simulink model "javi_FULL_model"  (R2023a)
settings: Solver=VariableStepAuto  StartTime=0.0  StopTime=0.5  RelTol=1e-3
undefined symbols (not defined in the file or in its folder): f_grid, L, R, tau, Vpeak_d1
libraries: spsControlledVoltageSourceLib x6, slpidlib x4, spsCurrentMeasurementLib x3, spsSeriesRLCBranchLib x3, powerlib_extras x1, spspowerguiLib x1
settings Model: Creator=citcea  LastModifiedBy=citcea

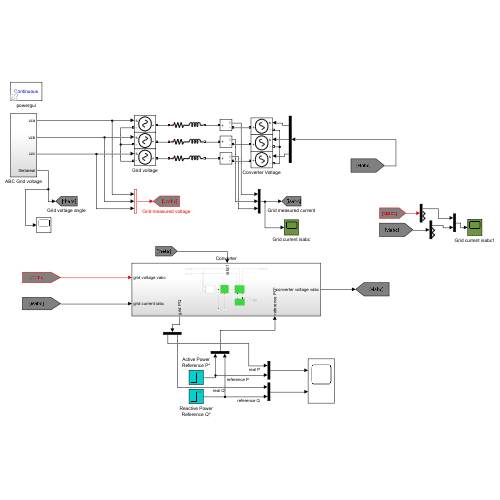
[thumbnail: Simulink's stored preview of the top-level diagram]
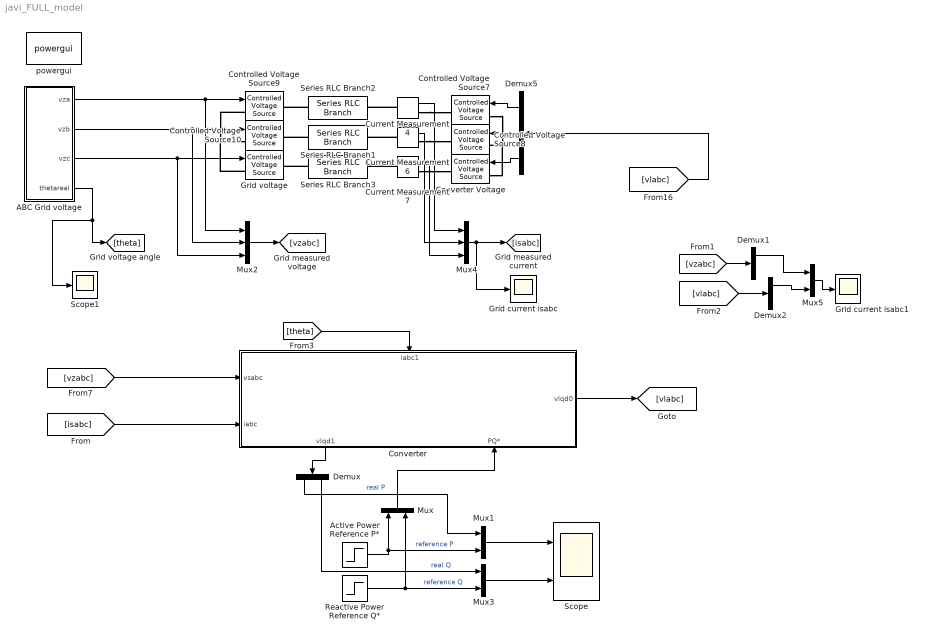
== system javi_FULL_model ==
  ABC Grid voltage : Subsystem
  Active Power Reference P* : Step  Time=0.1  After=100e6  SampleTime=0
  Controlled Voltage Source{7..10} (4 alike) : spsControlledVoltageSourceLib/Controlled Voltage Source  Initialize=off  Source_Type=AC  Amplitude=0  Phase=0  Frequency=0  Measurements=None
  Converter : Subsystem
      settings: PortSchema="{\"entries\":[{\"content\":{\"sides\":[{\"content\":{\"connectorIds\":[\"In1\",\"In2\"]},\"type\":\"ConnectorPlacement.EquallySpacedRectSide\",\"uuid\":\"584062e5-d349-4a6c-b774-2e2a2bb48d68\"},{\"content\":{\"connectorIds\":[\"Out1\"],\"side\":\"RIGHT\"},\"type\":\"ConnectorPlacement.EquallySpacedRectSide\",\"uuid\":\"a9b3d7e8-76a4-441e-96b8-94fa9e4298b7\"},{\"content\":{\"connectorIds\":[\"In3\"],\"side\":\"TOP\"},\"type\":\"ConnectorPlacement.EquallySpacedRectSide\",\"uuid\":\"fa132551-d5a3-4871-9f18-bb1732292fbb\"},{\"content\":{\"connectorIds\":[\"Out2\",\"In4\"],\"side\":\"BOTTOM\"},\"type\":\"ConnectorPlacement.EquallySpacedRectSide\",\"uuid\":\"9abb25d7-96ea-4765-9339-f819af1c9234\"}]},\"type\":\"ConnectorPlacement.EquallySpacedConnector\",\"uuid\":\"67c0bfb2-b216-417e-864f-4c59b5de7996\"}],\"packageUris\":[\"http://schema.mathworks.com/mf0/Connector/R2020b\"],\"version\":\"1.0\"}"
  Converter Voltage : spsControlledVoltageSourceLib/Controlled Voltage Source  Initialize=off  Source_Type=AC  Amplitude=0  Phase=0  Frequency=0  Measurements=None
  Current Measurement4 : spsCurrentMeasurementLib/Current Measurement  PhasorSimulation=off  OutputType=Complex  PSBequivalent=0
  Current Measurement6 : spsCurrentMeasurementLib/Current Measurement  PhasorSimulation=off  OutputType=Complex  PSBequivalent=0
  Current Measurement7 : spsCurrentMeasurementLib/Current Measurement  PhasorSimulation=off  OutputType=Complex  PSBequivalent=0
  Demux : Demux  Outputs=2
  Demux1 : Demux  Outputs=3
  Demux2 : Demux  Outputs=3
  Demux5 : Demux  Outputs=3
  Grid current isabc : Scope
  Grid current isabc1 : Scope
  Grid voltage : spsControlledVoltageSourceLib/Controlled Voltage Source  Initialize=off  Source_Type=AC  Amplitude=0  Phase=0  Frequency=0  Measurements=None
  Mux{,1,3,5} (4 alike) : Mux  Inputs=2
  Mux2 : Mux  Inputs=3
  Mux4 : Mux  Inputs=3
  Reactive Power Reference Q* : Step  Time=0.3  After=10e6  SampleTime=0
  Scope : Scope  NumInputPorts=2
  Scope1 : Scope
  Series RLC Branch1 : spsSeriesRLCBranchLib/Series RLC Branch  LConnTagsString=__new0  RConnTagsString=__new0  BranchType=RL  Resistance=R  Inductance=L  SetiL0=off  InitialCurrent=0  Capacitance=0  Setx0=off  InitialVoltage=0  Measurements=None
  Series RLC Branch2 : spsSeriesRLCBranchLib/Series RLC Branch  LConnTagsString=__new0  RConnTagsString=__new0  BranchType=RL  Resistance=R  Inductance=L  SetiL0=off  InitialCurrent=0  Capacitance=0  Setx0=off  InitialVoltage=0  Measurements=None
  Series RLC Branch3 : spsSeriesRLCBranchLib/Series RLC Branch  LConnTagsString=__new0  RConnTagsString=__new0  BranchType=RL  Resistance=R  Inductance=L  SetiL0=off  InitialCurrent=0  Capacitance=0  Setx0=off  InitialVoltage=0  Measurements=None
  powergui : spspowerguiLib/powergui  Priority=1  SimulationMode=Continuous  SampleTime=50e-6  frequency=60  Iterations=50  frequencyindice=0  Pbase=100e6  ErrMax=1e-4  UnitsV=kV  UnitsW=MW  buscounter=0  FunctionMessages=off  echomessages=off  EnableUseOfTLC=off  CurrentSourceSwitches=on  DisableSnubberDevices=off  DisableRonSwitches=off  DisableVfSwitches=off  DisplayEquations=off  AutomaticDiscreteSolvers=off  SolverType=Tustin  Interpol=off  ExternalGateDelay=off  methode=off  Ts=0  x0status=blocks  SPID=off  SwTol=0  HookPort=off  NonlinearTolerance=1e-4  nMaxIteration=100  ContinueOnMaxIteration=off  RestoreLinks=warning  ResistiveCurrentMeasurement=off  Frange=[0:2:500]  Ylog=off  Xlog=on  ShowGrid=off  save=off  variable=ZData  structure=0  ZoomFFT=off  StartTime=0.0  cycles=1  DisplayStyle=1  fundamental=60  FreqAxis=off  MaxFrequency=1000  frequencyindicesteady=1  RmsSteady=1  display=off
  wires:
  Mux2/1 -> [vzabc]
  Current Measurement4/1 -> Mux4/1
  Current Measurement6/1 -> Mux4/2
  Mux4/1 -> [isabc], Grid current isabc/1
  Current Measurement7/1 -> Mux4/3
  Demux5/3 -> Converter Voltage/1
  Demux5/1 -> Controlled Voltage Source7/1
  ABC Grid voltage/1(vza) -> Controlled Voltage Source9/1, Mux2/1
  ABC Grid voltage/2(vzb) -> Controlled Voltage Source10/1, Mux2/2
  ABC Grid voltage/3(vzc) -> Grid voltage/1, Mux2/3
  [vlabc] -> Demux5/1
  Demux5/2 -> Controlled Voltage Source8/1
  ABC Grid voltage/4(thetareal) -> Scope1/1, [theta]
  Converter/1(vlqd0) -> [vlabc]
  [isabc] -> Converter/2(iabc)
  [vzabc] -> Converter/1(vsabc)
  Mux/1 -> Converter/4(PQ*)
  Active Power Reference P*/1 -> Mux1/2, Mux/1  "reference P"
  Reactive Power Reference Q*/1 -> Mux3/2, Mux/2  "reference Q"
  Converter/2(vlqd1) -> Demux/1
  Demux/1 -> Mux1/1  "real P"
  Mux1/1 -> Scope/1
  Mux3/1 -> Scope/2
  Demux/2 -> Mux3/1  "real Q"
  [vzabc] -> Demux1/1
  [vlabc] -> Demux2/1
  Demux1/1 -> Mux5/1
  Mux5/1 -> Grid current isabc1/1
  Demux2/1 -> Mux5/2
  [theta] -> Converter/3(iabc1)
  connections:
  Grid voltage/LConn1 -- Controlled Voltage Source9/LConn1 -- Controlled Voltage Source10/LConn1
  Converter Voltage/LConn1 -- Controlled Voltage Source7/LConn1 -- Controlled Voltage Source8/LConn1
  Current Measurement4/LConn1 -- Series RLC Branch2/RConn1
  Series RLC Branch1/LConn1 -- Controlled Voltage Source10/RConn1
  Current Measurement6/RConn1 -- Controlled Voltage Source8/RConn1
  Current Measurement7/LConn1 -- Series RLC Branch3/RConn1
  Series RLC Branch2/LConn1 -- Controlled Voltage Source9/RConn1
  Current Measurement4/RConn1 -- Controlled Voltage Source7/RConn1
  Current Measurement6/LConn1 -- Series RLC Branch1/RConn1
  Current Measurement7/RConn1 -- Converter Voltage/RConn1
  Series RLC Branch3/LConn1 -- Grid voltage/RConn1

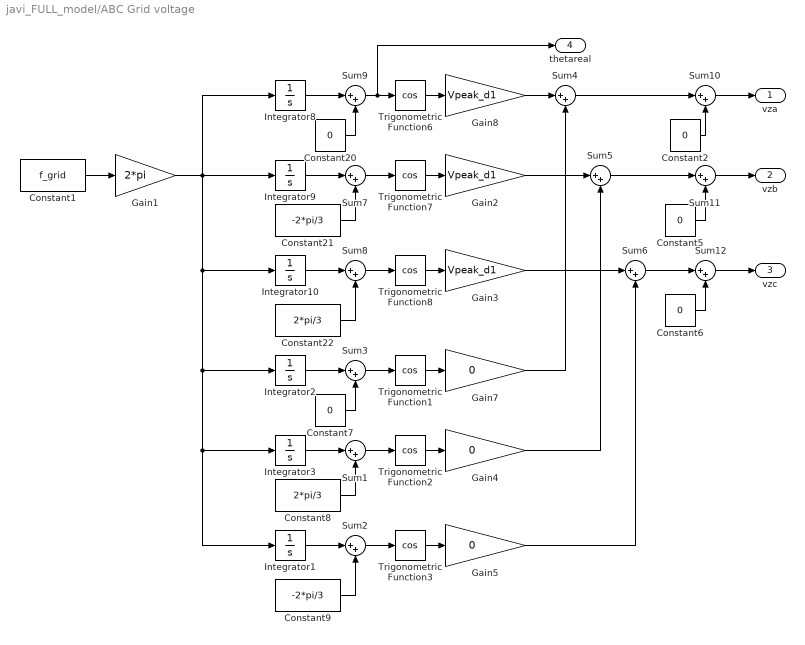
== system javi_FULL_model/ABC Grid voltage ==
  Constant1 : Constant  Value=f_grid
  Constant{2,5..7,20} (5 alike) : Constant  Value=0
  Constant21 : Constant  Value=-2*pi/3
  Constant22 : Constant  Value=2*pi/3
  Constant8 : Constant  Value=2*pi/3
  Constant9 : Constant  Value=-2*pi/3
  Gain1 : Gain  Gain=2*pi
  Gain2 : Gain  Gain=Vpeak_d1
  Gain3 : Gain  Gain=Vpeak_d1
  Gain4 : Gain  Gain=0
  Gain5 : Gain  Gain=0
  Gain7 : Gain  Gain=0
  Gain8 : Gain  Gain=Vpeak_d1
  Integrator{1..3,8..10} (6 alike) : Integrator
  Sum{1..12} (12 alike) : Sum  Inputs=|++
  Trigonometric Function{1..3,6..8} (6 alike) : Trigonometry  Operator=cos
  vza : Outport
  vzb : Outport  Port=2
  vzc : Outport  Port=3
  thetareal : Outport  Port=4
  wires:
  Sum12/1 -> vzc/1
  Sum11/1 -> vzb/1
  Sum10/1 -> vza/1
  Constant6/1 -> Sum12/2
  Constant5/1 -> Sum11/2
  Constant2/1 -> Sum10/2
  Sum6/1 -> Sum12/1
  Sum5/1 -> Sum11/1
  Sum4/1 -> Sum10/1
  Gain5/1 -> Sum6/2
  Gain4/1 -> Sum5/2
  Gain7/1 -> Sum4/2
  Trigonometric Function2/1 -> Gain4/1
  Trigonometric Function3/1 -> Gain5/1
  Sum3/1 -> Trigonometric Function1/1
  Constant9/1 -> Sum2/2
  Integrator1/1 -> Sum2/1
  Constant8/1 -> Sum1/2
  Integrator2/1 -> Sum3/1
  Gain1/1 -> Integrator9/1, Integrator8/1, Integrator10/1, Integrator2/1, Integrator1/1, Integrator3/1
  Sum1/1 -> Trigonometric Function2/1
  Constant7/1 -> Sum3/2
  Trigonometric Function1/1 -> Gain7/1
  Integrator3/1 -> Sum1/1
  Sum2/1 -> Trigonometric Function3/1
  Gain3/1 -> Sum6/1
  Gain2/1 -> Sum5/1
  Gain8/1 -> Sum4/1
  Trigonometric Function7/1 -> Gain2/1
  Trigonometric Function8/1 -> Gain3/1
  Constant1/1 -> Gain1/1
  Sum9/1 -> thetareal/1, Trigonometric Function6/1
  Constant22/1 -> Sum8/2
  Integrator10/1 -> Sum8/1
  Constant21/1 -> Sum7/2
  Integrator8/1 -> Sum9/1
  Sum7/1 -> Trigonometric Function7/1
  Constant20/1 -> Sum9/2
  Trigonometric Function6/1 -> Gain8/1
  Integrator9/1 -> Sum7/1
  Sum8/1 -> Trigonometric Function8/1

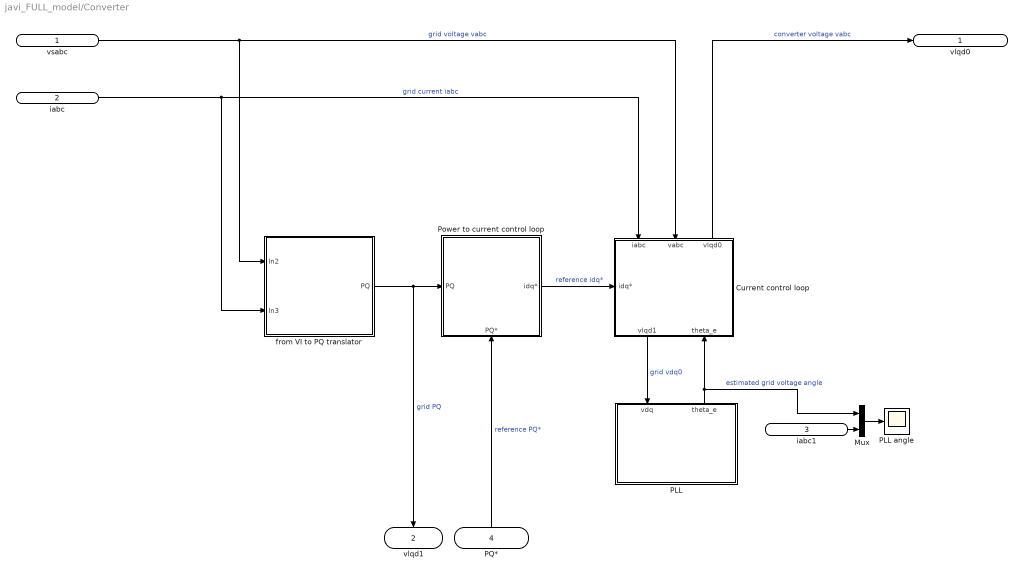
== system javi_FULL_model/Converter ==
  vsabc : Inport
  iabc : Inport  Port=2
  iabc1 : Inport  Port=3
  PQ* : Inport  Port=4
  Current control loop : Subsystem
      settings: PortSchema="{\"entries\":[{\"content\":{\"sides\":[{\"content\":{\"connectorIds\":[\"Out2\",\"In1\",\"In2\"]},\"type\":\"ConnectorPlacement.EquallySpacedRectSide\",\"uuid\":\"c04b464b-16ba-43bf-8c89-b835a7ede4b9\"},{\"content\":{\"connectorIds\":[\"In4\",\"Out1\"],\"side\":\"RIGHT\"},\"type\":\"ConnectorPlacement.EquallySpacedRectSide\",\"uuid\":\"740409c7-44aa-4313-af5e-f03563efb312\"},{\"content\":{\"side\":\"TOP\"},\"type\":\"ConnectorPlacement.EquallySpacedRectSide\",\"uuid\":\"d5fc34f0-88c0-4064-a212-e2f3525e0a41\"},{\"content\":{\"connectorIds\":[\"In3\"],\"side\":\"BOTTOM\"},\"type\":\"ConnectorPlacement.EquallySpacedRectSide\",\"uuid\":\"00c4ea66-ebf3-4884-86d2-74a5a00dfdcd\"}]},\"type\":\"ConnectorPlacement.EquallySpacedConnector\",\"uuid\":\"5b1879ce-fc34-4228-81c6-be4d14a0039a\"}],\"packageUris\":[\"http://schema.mathworks.com/mf0/Connector/R2020b\"],\"version\":\"1.0\"}"
  Mux : Mux  Inputs=2
  PLL : Subsystem
      settings: PortSchema="{\"entries\":[{\"content\":{\"sides\":[{\"content\":{\"connectorIds\":[\"Out1\",\"In1\"]},\"type\":\"ConnectorPlacement.EquallySpacedRectSide\",\"uuid\":\"1b368b75-2a8e-4f20-b703-977c9b032793\"},{\"content\":{\"side\":\"RIGHT\"},\"type\":\"ConnectorPlacement.EquallySpacedRectSide\",\"uuid\":\"82ee01ed-1d9e-40c1-8ec1-273e9e3bb456\"},{\"content\":{\"side\":\"TOP\"},\"type\":\"ConnectorPlacement.EquallySpacedRectSide\",\"uuid\":\"dfdc63e3-35c4-4b8d-aa5d-f501c13e42c1\"}]},\"type\":\"ConnectorPlacement.EquallySpacedConnector\",\"uuid\":\"13f018e6-0609-4dc5-a634-49aff68fea1b\"}],\"packageUris\":[\"http://schema.mathworks.com/mf0/Connector/R2020b\"],\"version\":\"1.0\"}"
  PLL angle : Scope
  Power to current control loop : Subsystem
      settings: PortSchema="{\"entries\":[{\"content\":{\"sides\":[{\"content\":{},\"type\":\"ConnectorPlacement.EquallySpacedRectSide\",\"uuid\":\"ef825e86-9abb-4c1d-b219-2a192ab282df\"},{\"content\":{\"connectorIds\":[\"In2\"],\"side\":\"RIGHT\"},\"type\":\"ConnectorPlacement.EquallySpacedRectSide\",\"uuid\":\"034459b8-9f08-4096-b542-16491f7ea4b2\"},{\"content\":{\"connectorIds\":[\"Out1\"],\"side\":\"TOP\"},\"type\":\"ConnectorPlacement.EquallySpacedRectSide\",\"uuid\":\"d0060c23-b394-4ccb-8e17-1dfe8e516f04\"},{\"content\":{\"connectorIds\":[\"In1\"],\"side\":\"BOTTOM\"},\"type\":\"ConnectorPlacement.EquallySpacedRectSide\",\"uuid\":\"50af44c6-d361-47aa-a23f-971b5daa1a8c\"}]},\"type\":\"ConnectorPlacement.EquallySpacedConnector\",\"uuid\":\"aefb8199-1196-4dbb-bffd-0cb2c3c781ab\"}],\"packageUris\":[\"http://schema.mathworks.com/mf0/Connector/R2020b\"],\"version\":\"1.0\"}"
  from VI to PQ translator : Subsystem
  vlqd0 : Outport
  vlqd1 : Outport  Port=2
  wires:
  vsabc/1 -> Current control loop/1(vabc), from VI to PQ translator/1(In2)  "grid voltage vabc"
  iabc/1 -> Current control loop/2(iabc), from VI to PQ translator/2(In3)  "grid current iabc"
  Current control loop/2(vlqd0) -> vlqd0/1  "converter voltage vabc"
  PLL/1(theta_e) -> Mux/1, Current control loop/4(theta_e)  "estimated grid voltage angle"
  Power to current control loop/1(idq*) -> Current control loop/3(idq*)  "reference idq*"
  PQ*/1 -> Power to current control loop/2(PQ*)  "reference PQ*"
  from VI to PQ translator/1(PQ) -> Power to current control loop/1(PQ), vlqd1/1  "grid PQ"
  Current control loop/1(vlqd1) -> PLL/1(vdq)  "grid vdq0"
  iabc1/1 -> Mux/2
  Mux/1 -> PLL angle/1

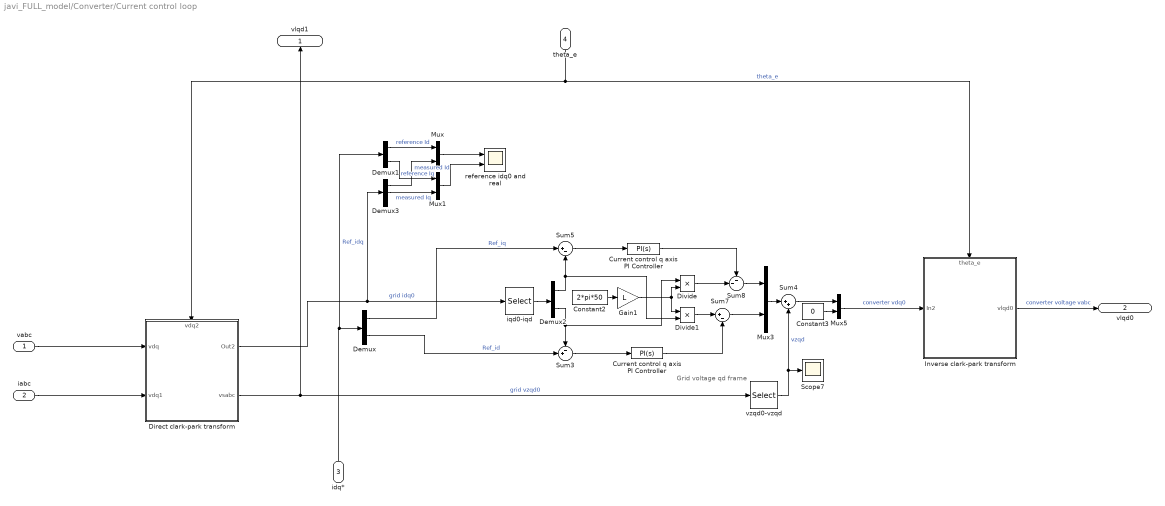
== system javi_FULL_model/Converter/Current control loop ==
  note: Grid voltage qd frame
  vabc : Inport
  iabc : Inport  Port=2
  idq* : Inport  Port=3
  theta_e : Inport  Port=4
  Constant2 : Constant  Value=2*pi*50  SampleTime=-1
  Constant3 : Constant  Value=0
  Current control q axis PI Controller : slpidlib/PID Controller  Controller=PI  Form=Parallel  TimeDomain=Continuous-time  UseExternalTs=off  SampleTime=1  IntegratorMethod=Forward Euler  FilterMethod=Forward Euler  ControllerParametersSource=internal  P=L/tau  I=R/tau  UseKiTs=off  D=0  N=100  UseFilter=on  TunerSelectOption=Transfer Function Based (PID Tuner App)  InitialConditionSource=internal  InitialConditionForIntegrator=0  InitialConditionForFilter=0  DifferentiatorICPrevScaledInput=0  ExternalReset=none  TrackingMode=off  Kt=1  LimitOutput=off  SatLimitsSource=internal  UpperSaturationLimit=inf  LowerSaturationLimit=-inf  LinearizeAsGain=on  AntiWindupMode=none  Kb=1  LimitIntegrator=off  UpperIntegratorSaturationLimit=inf  LowerIntegratorSaturationLimit=-inf  POutMin=[]  POutMax=[]  IOutMin=[]  IOutMax=[]  DOutMin=[]  DOutMax=[]  NOutMin=[]  NOutMax=[]  SumOutMin=[]  SumOutMax=[]  SaturationOutMin=[]  SaturationOutMax=[]  PParamMin=[]  PParamMax=[]  IParamMin=[]  IParamMax=[]  DParamMin=[]  DParamMax=[]  NParamMin=[]  NParamMax=[]  KbParamMin=[]  KbParamMax=[]  KtParamMin=[]  KtParamMax=[]  KbOutMin=[]  KbOutMax=[]  KtOutMin=[]  KtOutMax=[]  IntegratorOutMin=[]  IntegratorOutMax=[]  FilterOutMin=[]  FilterOutMax=[]  SumI1OutMin=[]  SumI1OutMax=[]  SumI2OutMin=[]  SumI2OutMax=[]  SumI3OutMin=[]  SumI3OutMax=[]  SumI4OutMin=[]  SumI4OutMax=[]  SumDOutMin=[]  SumDOutMax=[]  DifferentiatorOutMin=[]  DifferentiatorOutMax=[]  FilterDiffOutCoefMin=[]  FilterDiffOutCoefMax=[]  ReciprocalOutMin=[]  ReciprocalOutMax=[]  SumDenOutMin=[]  SumDenOutMax=[]  SumNumOutMin=[]  SumNumOutMax=[]  DivideOutMin=[]  DivideOutMax=[]  UdiffTsProdOutMin=[]  UdiffTsProdOutMax=[]  NTsProdOutMin=[]  NTsProdOutMax=[]  UintegralTsProdOutMin=[]  UintegralTsProdOutMax=[]  UngainTsProdOutMin=[]  UngainTsProdOutMax=[]  ClampingZeroOutDataTypeStr=Inherit: Inherit via back propagation  ClampingZeroOutMin=[]  ClampingZeroOutMax=[]  FilterDenConstantOutDataTypeStr=Inherit: Inherit via back propagation  FilterDenConstantOutMin=[]  FilterDenConstantOutMax=[]  PCopyOutDataTypeStr=Inherit: Inherit via back propagation  PCopyOutMin=[]  PCopyOutMax=[]  NCopyOutDataTypeStr=Inherit: Inherit via back propagation  NCopyOutMin=[]  NCopyOutMax=[]  IntegratorContinuousStateAttributes=''  IntegratorStateMustResolveToSignalObject=off  IntegratorRTWStateStorageClass=Auto  FilterContinuousStateAttributes=''  FilterStateMustResolveToSignalObject=off  FilterRTWStateStorageClass=Auto  ParallelPVariant=InternalParameters  IdealPVariant=Disabled  IVariant=InternalParameters  DVariant=Disabled  IntegratorVariant=Continuous  SatVariant=Disabled  AWVariant=Passthrough  PCopyVariant=Disabled  TRVariant=Disabled  FdbkBlocksVariant=Forward  IdealPFdbkVariant=Disabled  SatFdbkVariant=Disabled  DerivativeFilterVariant=Disabled  NVariant=Disabled  NCopyVariant=Disabled_SignalSpec  FilterICVariant=Disabled  IntegratorICVariant=InternalICs  ExternalResetVariant=Disabled  TRSumVariant=Passthrough  SumFdbkVariant=Disabled  SumVariant=Sum_PI  TsampFilterVariant=InternalTs  TsampNgainVariant=Passthrough  TsampIntegralVariant=Disabled_SignalSpec  ExternalSaturationOutDataTypeStr=Inherit: Same as second input
  "Current control q axis PI Controller " : slpidlib/PID Controller  Controller=PI  Form=Parallel  TimeDomain=Continuous-time  UseExternalTs=off  SampleTime=1  IntegratorMethod=Forward Euler  FilterMethod=Forward Euler  ControllerParametersSource=internal  P=L/tau  I=R/tau  UseKiTs=off  D=0  N=100  UseFilter=on  TunerSelectOption=Transfer Function Based (PID Tuner App)  InitialConditionSource=internal  InitialConditionForIntegrator=0  InitialConditionForFilter=0  DifferentiatorICPrevScaledInput=0  ExternalReset=none  TrackingMode=off  Kt=1  LimitOutput=off  SatLimitsSource=internal  UpperSaturationLimit=inf  LowerSaturationLimit=-inf  LinearizeAsGain=on  AntiWindupMode=none  Kb=1  LimitIntegrator=off  UpperIntegratorSaturationLimit=inf  LowerIntegratorSaturationLimit=-inf  POutMin=[]  POutMax=[]  IOutMin=[]  IOutMax=[]  DOutMin=[]  DOutMax=[]  NOutMin=[]  NOutMax=[]  SumOutMin=[]  SumOutMax=[]  SaturationOutMin=[]  SaturationOutMax=[]  PParamMin=[]  PParamMax=[]  IParamMin=[]  IParamMax=[]  DParamMin=[]  DParamMax=[]  NParamMin=[]  NParamMax=[]  KbParamMin=[]  KbParamMax=[]  KtParamMin=[]  KtParamMax=[]  KbOutMin=[]  KbOutMax=[]  KtOutMin=[]  KtOutMax=[]  IntegratorOutMin=[]  IntegratorOutMax=[]  FilterOutMin=[]  FilterOutMax=[]  SumI1OutMin=[]  SumI1OutMax=[]  SumI2OutMin=[]  SumI2OutMax=[]  SumI3OutMin=[]  SumI3OutMax=[]  SumI4OutMin=[]  SumI4OutMax=[]  SumDOutMin=[]  SumDOutMax=[]  DifferentiatorOutMin=[]  DifferentiatorOutMax=[]  FilterDiffOutCoefMin=[]  FilterDiffOutCoefMax=[]  ReciprocalOutMin=[]  ReciprocalOutMax=[]  SumDenOutMin=[]  SumDenOutMax=[]  SumNumOutMin=[]  SumNumOutMax=[]  DivideOutMin=[]  DivideOutMax=[]  UdiffTsProdOutMin=[]  UdiffTsProdOutMax=[]  NTsProdOutMin=[]  NTsProdOutMax=[]  UintegralTsProdOutMin=[]  UintegralTsProdOutMax=[]  UngainTsProdOutMin=[]  UngainTsProdOutMax=[]  ClampingZeroOutDataTypeStr=Inherit: Inherit via back propagation  ClampingZeroOutMin=[]  ClampingZeroOutMax=[]  FilterDenConstantOutDataTypeStr=Inherit: Inherit via back propagation  FilterDenConstantOutMin=[]  FilterDenConstantOutMax=[]  PCopyOutDataTypeStr=Inherit: Inherit via back propagation  PCopyOutMin=[]  PCopyOutMax=[]  NCopyOutDataTypeStr=Inherit: Inherit via back propagation  NCopyOutMin=[]  NCopyOutMax=[]  IntegratorContinuousStateAttributes=''  IntegratorStateMustResolveToSignalObject=off  IntegratorRTWStateStorageClass=Auto  FilterContinuousStateAttributes=''  FilterStateMustResolveToSignalObject=off  FilterRTWStateStorageClass=Auto  ParallelPVariant=InternalParameters  IdealPVariant=Disabled  IVariant=InternalParameters  DVariant=Disabled  IntegratorVariant=Continuous  SatVariant=Disabled  AWVariant=Passthrough  PCopyVariant=Disabled  TRVariant=Disabled  FdbkBlocksVariant=Forward  IdealPFdbkVariant=Disabled  SatFdbkVariant=Disabled  DerivativeFilterVariant=Disabled  NVariant=Disabled  NCopyVariant=Disabled_SignalSpec  FilterICVariant=Disabled  IntegratorICVariant=InternalICs  ExternalResetVariant=Disabled  TRSumVariant=Passthrough  SumFdbkVariant=Disabled  SumVariant=Sum_PI  TsampFilterVariant=InternalTs  TsampNgainVariant=Passthrough  TsampIntegralVariant=Disabled_SignalSpec  ExternalSaturationOutDataTypeStr=Inherit: Same as second input
  Demux : Demux  Outputs=2
  Demux1 : Demux  Outputs=2
  Demux2 : Demux  Outputs=2
  Demux3 : Demux  Outputs=3
  Direct clark-park transform : Subsystem
      settings: PortSchema="{\"entries\":[{\"content\":{\"sides\":[{\"content\":{\"connectorIds\":[\"In1\",\"In2\"]},\"type\":\"ConnectorPlacement.EquallySpacedRectSide\",\"uuid\":\"fbcb26c8-642f-4dfe-8454-ba7bccc8a058\"},{\"content\":{\"connectorIds\":[\"Out1\",\"Out2\"],\"side\":\"RIGHT\"},\"type\":\"ConnectorPlacement.EquallySpacedRectSide\",\"uuid\":\"4c408f54-c932-4abe-8c91-a3cf5cf07aa2\"},{\"content\":{\"connectorIds\":[\"In3\"],\"side\":\"TOP\"},\"type\":\"ConnectorPlacement.EquallySpacedRectSide\",\"uuid\":\"ce403afa-f5e3-434a-92aa-74c44e817e3e\"}]},\"type\":\"ConnectorPlacement.EquallySpacedConnector\",\"uuid\":\"c9773e31-1609-4d99-a6b0-abdbc446c6a8\"}],\"packageUris\":[\"http://schema.mathworks.com/mf0/Connector/R2020b\"],\"version\":\"1.0\"}"
  Divide : Product  Inputs=**
  Divide1 : Product  Inputs=**
  Gain1 : Gain  Gain=L
  Inverse clark-park transform : Subsystem
      settings: PortSchema="{\"entries\":[{\"content\":{\"sides\":[{\"content\":{\"connectorIds\":[\"In1\"]},\"type\":\"ConnectorPlacement.EquallySpacedRectSide\",\"uuid\":\"fbcb26c8-642f-4dfe-8454-ba7bccc8a058\"},{\"content\":{\"connectorIds\":[\"Out1\"],\"side\":\"RIGHT\"},\"type\":\"ConnectorPlacement.EquallySpacedRectSide\",\"uuid\":\"4c408f54-c932-4abe-8c91-a3cf5cf07aa2\"},{\"content\":{\"connectorIds\":[\"In2\"],\"side\":\"TOP\"},\"type\":\"ConnectorPlacement.EquallySpacedRectSide\",\"uuid\":\"ce403afa-f5e3-434a-92aa-74c44e817e3e\"}]},\"type\":\"ConnectorPlacement.EquallySpacedConnector\",\"uuid\":\"c9773e31-1609-4d99-a6b0-abdbc446c6a8\"}],\"packageUris\":[\"http://schema.mathworks.com/mf0/Connector/R2020b\"],\"version\":\"1.0\"}"
  Mux{,1,3,5} (4 alike) : Mux  Inputs=2
  Scope7 : Scope
  Sum3 : Sum  Inputs=-+|
  Sum4 : Sum  Inputs=|++
  Sum5 : Sum  Inputs=|+-
  Sum7 : Sum  Inputs=|+-
  Sum8 : Sum  Inputs=--|
  iqd0-iqd : Selector  InputPortWidth=3  IndexOptions=Index vector (dialog)  Indices=[1 2]  OutputSizes=1
  reference idq0 and real : Scope  NumInputPorts=2
  vzqd0-vzqd : Selector  InputPortWidth=3  IndexOptions=Index vector (dialog)  Indices=[1 2]  OutputSizes=1
  vlqd1 : Outport
  vlqd0 : Outport  Port=2
  wires:
  Direct clark-park transform/1(Out2) -> Demux3/1, iqd0-iqd/1  "grid idq0"
  Mux5/1 -> Inverse clark-park transform/1(In2)  "converter vdq0"
  idq*/1 -> Demux1/1, Demux/1  "Ref_idq"
  Current control q axis PI Controller/1 -> Sum8/1
  Demux/2 -> Sum3/2  "Ref_id"
  iqd0-iqd/1 -> Demux2/1
  Direct clark-park transform/2(vsabc) -> vzqd0-vzqd/1, vlqd1/1  "grid vzqd0"
  Divide/1 -> Sum8/2
  Demux2/2 -> Sum3/1, Divide/1
  Demux2/1 -> Divide1/2, Sum5/2
  Constant3/1 -> Mux5/2
  Sum8/1 -> Mux3/1
  "Current control q axis PI Controller "/1 -> Sum7/2
  Sum4/1 -> Mux5/1
  Constant2/1 -> Gain1/1
  Sum5/1 -> Current control q axis PI Controller/1
  vzqd0-vzqd/1 -> Scope7/1, Sum4/2  "vzqd"
  Demux/1 -> Sum5/1  "Ref_iq"
  Mux3/1 -> Sum4/1
  Divide1/1 -> Sum7/1
  Sum3/1 -> "Current control q axis PI Controller "/1
  Gain1/1 -> Divide1/1, Divide/2
  Sum7/1 -> Mux3/2
  Inverse clark-park transform/1(vlqd0) -> vlqd0/1  "converter voltage vabc"
  vabc/1 -> Direct clark-park transform/1(vdq)
  iabc/1 -> Direct clark-park transform/2(vdq1)
  theta_e/1 -> Direct clark-park transform/3(vdq2), Inverse clark-park transform/2(theta_e)  "theta_e"
  Demux1/1 -> Mux/1  "reference Id"
  Mux/1 -> reference idq0 and real/1
  Demux3/1 -> Mux/2  "measured Id"
  Demux1/2 -> Mux1/1  "reference Iq"
  Demux3/2 -> Mux1/2  "measured Iq"
  Mux1/1 -> reference idq0 and real/2

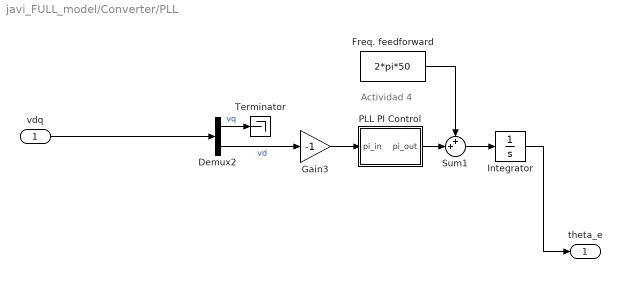
== system javi_FULL_model/Converter/PLL ==
  note: Actividad 4
  vdq : Inport
  Demux2 : Demux  Outputs=2
  Freq. feedforward : Constant  Value=2*pi*50
  Gain3 : Gain  Gain=-1
  Integrator : Integrator
  PLL PI Control : Subsystem
  Sum1 : Sum  Inputs=++|
  Terminator : Terminator
  theta_e : Outport
  wires:
  Gain3/1 -> PLL PI Control/1(pi_in)
  Demux2/1 -> Terminator/1  "vq"
  Integrator/1 -> theta_e/1
  vdq/1 -> Demux2/1
  Sum1/1 -> Integrator/1
  PLL PI Control/1(pi_out) -> Sum1/2
  Freq. feedforward/1 -> Sum1/1
  Demux2/2 -> Gain3/1  "vd"

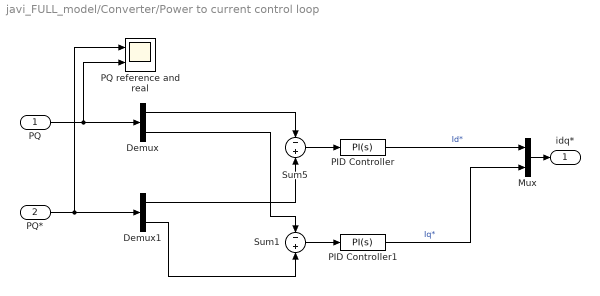
== system javi_FULL_model/Converter/Power to current control loop ==
  PQ : Inport
  PQ* : Inport  Port=2
  Demux : Demux  Outputs=2
  Demux1 : Demux  Outputs=2
  Mux : Mux  Inputs=2
  PID Controller : slpidlib/PID Controller  Controller=PI  Form=Parallel  TimeDomain=Continuous-time  UseExternalTs=off  SampleTime=1  IntegratorMethod=Forward Euler  FilterMethod=Forward Euler  ControllerParametersSource=internal  P=7.5e-7  I=1.2e-04  UseKiTs=off  D=0  N=100  UseFilter=on  TunerSelectOption=Transfer Function Based (PID Tuner App)  InitialConditionSource=internal  InitialConditionForIntegrator=0  InitialConditionForFilter=0  DifferentiatorICPrevScaledInput=0  ExternalReset=none  TrackingMode=off  Kt=1  LimitOutput=off  SatLimitsSource=internal  UpperSaturationLimit=inf  LowerSaturationLimit=-inf  LinearizeAsGain=on  AntiWindupMode=none  Kb=1  LimitIntegrator=off  UpperIntegratorSaturationLimit=inf  LowerIntegratorSaturationLimit=-inf  POutMin=[]  POutMax=[]  IOutMin=[]  IOutMax=[]  DOutMin=[]  DOutMax=[]  NOutMin=[]  NOutMax=[]  SumOutMin=[]  SumOutMax=[]  SaturationOutMin=[]  SaturationOutMax=[]  PParamMin=[]  PParamMax=[]  IParamMin=[]  IParamMax=[]  DParamMin=[]  DParamMax=[]  NParamMin=[]  NParamMax=[]  KbParamMin=[]  KbParamMax=[]  KtParamMin=[]  KtParamMax=[]  KbOutMin=[]  KbOutMax=[]  KtOutMin=[]  KtOutMax=[]  IntegratorOutMin=[]  IntegratorOutMax=[]  FilterOutMin=[]  FilterOutMax=[]  SumI1OutMin=[]  SumI1OutMax=[]  SumI2OutMin=[]  SumI2OutMax=[]  SumI3OutMin=[]  SumI3OutMax=[]  SumI4OutMin=[]  SumI4OutMax=[]  SumDOutMin=[]  SumDOutMax=[]  DifferentiatorOutMin=[]  DifferentiatorOutMax=[]  FilterDiffOutCoefMin=[]  FilterDiffOutCoefMax=[]  ReciprocalOutMin=[]  ReciprocalOutMax=[]  SumDenOutMin=[]  SumDenOutMax=[]  SumNumOutMin=[]  SumNumOutMax=[]  DivideOutMin=[]  DivideOutMax=[]  UdiffTsProdOutMin=[]  UdiffTsProdOutMax=[]  NTsProdOutMin=[]  NTsProdOutMax=[]  UintegralTsProdOutMin=[]  UintegralTsProdOutMax=[]  UngainTsProdOutMin=[]  UngainTsProdOutMax=[]  ClampingZeroOutDataTypeStr=Inherit: Inherit via back propagation  ClampingZeroOutMin=[]  ClampingZeroOutMax=[]  FilterDenConstantOutDataTypeStr=Inherit: Inherit via back propagation  FilterDenConstantOutMin=[]  FilterDenConstantOutMax=[]  PCopyOutDataTypeStr=Inherit: Inherit via back propagation  PCopyOutMin=[]  PCopyOutMax=[]  NCopyOutDataTypeStr=Inherit: Inherit via back propagation  NCopyOutMin=[]  NCopyOutMax=[]  IntegratorContinuousStateAttributes=''  IntegratorStateMustResolveToSignalObject=off  IntegratorRTWStateStorageClass=Auto  FilterContinuousStateAttributes=''  FilterStateMustResolveToSignalObject=off  FilterRTWStateStorageClass=Auto  ParallelPVariant=InternalParameters  IdealPVariant=Disabled  IVariant=InternalParameters  DVariant=Disabled  IntegratorVariant=Continuous  SatVariant=Disabled  AWVariant=Passthrough  PCopyVariant=Disabled  TRVariant=Disabled  FdbkBlocksVariant=Forward  IdealPFdbkVariant=Disabled  SatFdbkVariant=Disabled  DerivativeFilterVariant=Disabled  NVariant=Disabled  NCopyVariant=Disabled_SignalSpec  FilterICVariant=Disabled  IntegratorICVariant=InternalICs  ExternalResetVariant=Disabled  TRSumVariant=Passthrough  SumFdbkVariant=Disabled  SumVariant=Sum_PI  TsampFilterVariant=InternalTs  TsampNgainVariant=Passthrough  TsampIntegralVariant=Disabled_SignalSpec  ExternalSaturationOutDataTypeStr=Inherit: Same as second input
  PID Controller1 : slpidlib/PID Controller  Controller=PI  Form=Parallel  TimeDomain=Continuous-time  UseExternalTs=off  SampleTime=1  IntegratorMethod=Forward Euler  FilterMethod=Forward Euler  ControllerParametersSource=internal  P=7.2e-6  I=2.35e-04  UseKiTs=off  D=0  N=100  UseFilter=on  TunerSelectOption=Transfer Function Based (PID Tuner App)  InitialConditionSource=internal  InitialConditionForIntegrator=0  InitialConditionForFilter=0  DifferentiatorICPrevScaledInput=0  ExternalReset=none  TrackingMode=off  Kt=1  LimitOutput=off  SatLimitsSource=internal  UpperSaturationLimit=inf  LowerSaturationLimit=-inf  LinearizeAsGain=on  AntiWindupMode=none  Kb=1  LimitIntegrator=off  UpperIntegratorSaturationLimit=inf  LowerIntegratorSaturationLimit=-inf  POutMin=[]  POutMax=[]  IOutMin=[]  IOutMax=[]  DOutMin=[]  DOutMax=[]  NOutMin=[]  NOutMax=[]  SumOutMin=[]  SumOutMax=[]  SaturationOutMin=[]  SaturationOutMax=[]  PParamMin=[]  PParamMax=[]  IParamMin=[]  IParamMax=[]  DParamMin=[]  DParamMax=[]  NParamMin=[]  NParamMax=[]  KbParamMin=[]  KbParamMax=[]  KtParamMin=[]  KtParamMax=[]  KbOutMin=[]  KbOutMax=[]  KtOutMin=[]  KtOutMax=[]  IntegratorOutMin=[]  IntegratorOutMax=[]  FilterOutMin=[]  FilterOutMax=[]  SumI1OutMin=[]  SumI1OutMax=[]  SumI2OutMin=[]  SumI2OutMax=[]  SumI3OutMin=[]  SumI3OutMax=[]  SumI4OutMin=[]  SumI4OutMax=[]  SumDOutMin=[]  SumDOutMax=[]  DifferentiatorOutMin=[]  DifferentiatorOutMax=[]  FilterDiffOutCoefMin=[]  FilterDiffOutCoefMax=[]  ReciprocalOutMin=[]  ReciprocalOutMax=[]  SumDenOutMin=[]  SumDenOutMax=[]  SumNumOutMin=[]  SumNumOutMax=[]  DivideOutMin=[]  DivideOutMax=[]  UdiffTsProdOutMin=[]  UdiffTsProdOutMax=[]  NTsProdOutMin=[]  NTsProdOutMax=[]  UintegralTsProdOutMin=[]  UintegralTsProdOutMax=[]  UngainTsProdOutMin=[]  UngainTsProdOutMax=[]  ClampingZeroOutDataTypeStr=Inherit: Inherit via back propagation  ClampingZeroOutMin=[]  ClampingZeroOutMax=[]  FilterDenConstantOutDataTypeStr=Inherit: Inherit via back propagation  FilterDenConstantOutMin=[]  FilterDenConstantOutMax=[]  PCopyOutDataTypeStr=Inherit: Inherit via back propagation  PCopyOutMin=[]  PCopyOutMax=[]  NCopyOutDataTypeStr=Inherit: Inherit via back propagation  NCopyOutMin=[]  NCopyOutMax=[]  IntegratorContinuousStateAttributes=''  IntegratorStateMustResolveToSignalObject=off  IntegratorRTWStateStorageClass=Auto  FilterContinuousStateAttributes=''  FilterStateMustResolveToSignalObject=off  FilterRTWStateStorageClass=Auto  ParallelPVariant=InternalParameters  IdealPVariant=Disabled  IVariant=InternalParameters  DVariant=Disabled  IntegratorVariant=Continuous  SatVariant=Disabled  AWVariant=Passthrough  PCopyVariant=Disabled  TRVariant=Disabled  FdbkBlocksVariant=Forward  IdealPFdbkVariant=Disabled  SatFdbkVariant=Disabled  DerivativeFilterVariant=Disabled  NVariant=Disabled  NCopyVariant=Disabled_SignalSpec  FilterICVariant=Disabled  IntegratorICVariant=InternalICs  ExternalResetVariant=Disabled  TRSumVariant=Passthrough  SumFdbkVariant=Disabled  SumVariant=Sum_PI  TsampFilterVariant=InternalTs  TsampNgainVariant=Passthrough  TsampIntegralVariant=Disabled_SignalSpec  ExternalSaturationOutDataTypeStr=Inherit: Same as second input
  PQ reference and real : Scope  NumInputPorts=2
  Sum1 : Sum  Inputs=-+
  Sum5 : Sum  Inputs=-+
  idq* : Outport
  wires:
  Sum5/1 -> PID Controller/1
  PID Controller/1 -> Mux/1  "Id*"
  PID Controller1/1 -> Mux/2  "Iq*"
  Sum1/1 -> PID Controller1/1
  PQ/1 -> PQ reference and real/2, Demux/1
  PQ*/1 -> PQ reference and real/1, Demux1/1
  Demux/1 -> Sum5/1
  Demux1/1 -> Sum5/2
  Demux/2 -> Sum1/1
  Demux1/2 -> Sum1/2
  Mux/1 -> idq*/1

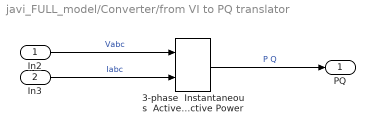
== system javi_FULL_model/Converter/from VI to PQ translator ==
  In2 : Inport
  In3 : Inport  Port=2
  3-phase  Instantaneous  Active & Reactive Power : powerlib_extras/Measurements/3-phase  Instantaneous  Active & Reactive Power
  PQ : Outport
  wires:
  In3/1 -> 3-phase  Instantaneous  Active & Reactive Power/2  "Iabc"
  3-phase  Instantaneous  Active & Reactive Power/1 -> PQ/1  "P Q"
  In2/1 -> 3-phase  Instantaneous  Active & Reactive Power/1  "Vabc"

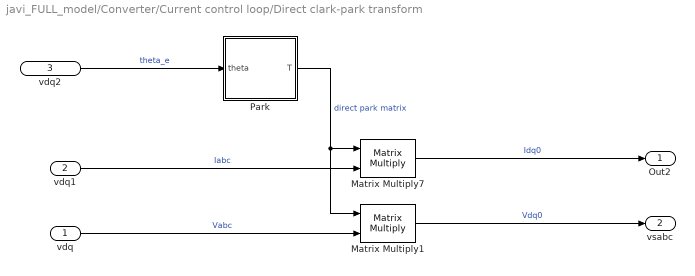
== system javi_FULL_model/Converter/Current control loop/Direct clark-park transform ==
  vdq : Inport
  vdq1 : Inport  Port=2
  vdq2 : Inport  Port=3
  Matrix Multiply1 : Product  Multiplication=Matrix(*)
  Matrix Multiply7 : Product  Multiplication=Matrix(*)
  Park : Subsystem
  Out2 : Outport
  vsabc : Outport  Port=2
  wires:
  vdq2/1 -> Park/1(theta)  "theta_e"
  vdq1/1 -> Matrix Multiply7/2  "Iabc"
  Park/1(T) -> Matrix Multiply1/1, Matrix Multiply7/1  "direct park matrix"
  vdq/1 -> Matrix Multiply1/2  "Vabc"
  Matrix Multiply1/1 -> vsabc/1  "Vdq0"
  Matrix Multiply7/1 -> Out2/1  "Idq0"

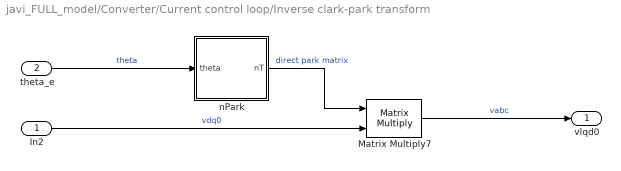
== system javi_FULL_model/Converter/Current control loop/Inverse clark-park transform ==
  In2 : Inport
  theta_e : Inport  Port=2
  Matrix Multiply7 : Product  Multiplication=Matrix(*)
  nPark : Subsystem
  vlqd0 : Outport
  wires:
  theta_e/1 -> nPark/1(theta)  "theta"
  nPark/1("nT ") -> Matrix Multiply7/1  "direct park matrix"
  Matrix Multiply7/1 -> vlqd0/1  "vabc"
  In2/1 -> Matrix Multiply7/2  "vdq0"

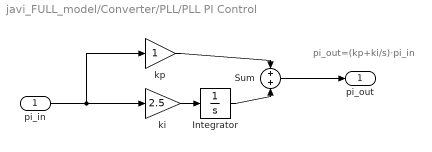
== system javi_FULL_model/Converter/PLL/PLL PI Control ==
  note: pi_out=(kp+ki/s)·pi_in
  pi_in : Inport
  Integrator : Integrator
  Sum : Sum
  ki : Gain  Gain=2.5
  kp : Gain
  pi_out : Outport
  wires:
  Sum/1 -> pi_out/1
  Integrator/1 -> Sum/2
  ki/1 -> Integrator/1
  kp/1 -> Sum/1
  pi_in/1 -> ki/1, kp/1

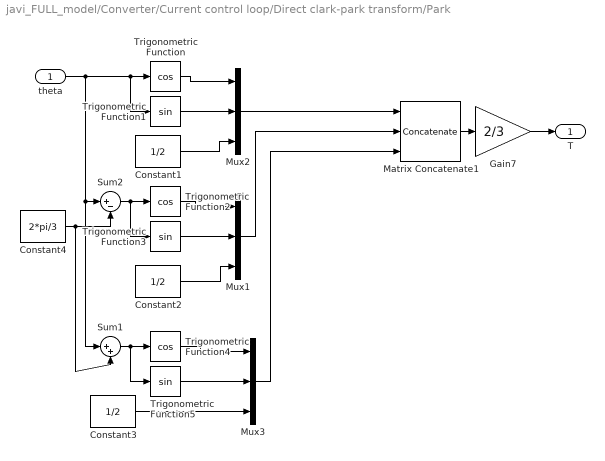
== system javi_FULL_model/Converter/Current control loop/Direct clark-park transform/Park ==
  theta : Inport
  Constant1 : Constant  Value=1/2  SampleTime=0
  Constant2 : Constant  Value=1/2  SampleTime=0
  Constant3 : Constant  Value=1/2  SampleTime=0
  Constant4 : Constant  Value=2*pi/3  SampleTime=0
  Gain7 : Gain  Gain=2/3
  Matrix Concatenate1 : Concatenate  NumInputs=3  Mode=Multidimensional array  ConcatenateDimension=2
  Mux1 : Mux  Inputs=3
  Mux2 : Mux  Inputs=3
  Mux3 : Mux  Inputs=3
  Sum1 : Sum  Inputs=|++
  Sum2 : Sum  Inputs=|+-
  Trigonometric Function : Trigonometry  Operator=cos
  Trigonometric Function1 : Trigonometry
  Trigonometric Function2 : Trigonometry  Operator=cos
  Trigonometric Function3 : Trigonometry
  Trigonometric Function4 : Trigonometry  Operator=cos
  Trigonometric Function5 : Trigonometry
  T : Outport
  wires:
  Gain7/1 -> T/1
  theta/1 -> Trigonometric Function1/1, Trigonometric Function/1, Sum2/1, Sum1/1
  Matrix Concatenate1/1 -> Gain7/1
  Mux3/1 -> Matrix Concatenate1/3
  Mux1/1 -> Matrix Concatenate1/2
  Mux2/1 -> Matrix Concatenate1/1
  Trigonometric Function5/1 -> Mux3/2
  Trigonometric Function4/1 -> Mux3/1
  Trigonometric Function3/1 -> Mux1/2
  Trigonometric Function2/1 -> Mux1/1
  Trigonometric Function1/1 -> Mux2/2
  Trigonometric Function/1 -> Mux2/1
  Constant4/1 -> Sum1/2, Sum2/2
  Sum1/1 -> Trigonometric Function5/1, Trigonometric Function4/1
  Sum2/1 -> Trigonometric Function3/1, Trigonometric Function2/1
  Constant1/1 -> Mux2/3
  Constant2/1 -> Mux1/3
  Constant3/1 -> Mux3/3

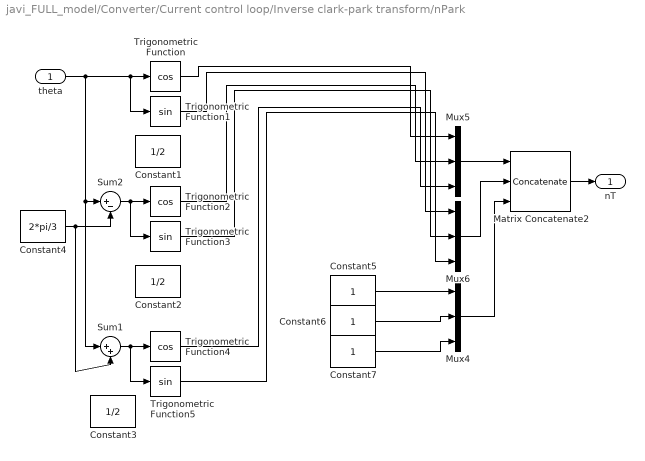
== system javi_FULL_model/Converter/Current control loop/Inverse clark-park transform/nPark ==
  theta : Inport
  Constant1 : Constant  Value=1/2  SampleTime=0
  Constant2 : Constant  Value=1/2  SampleTime=0
  Constant3 : Constant  Value=1/2  SampleTime=0
  Constant4 : Constant  Value=2*pi/3  SampleTime=0
  Constant5 : Constant  SampleTime=0
  Constant6 : Constant  SampleTime=0
  Constant7 : Constant  SampleTime=0
  Matrix Concatenate2 : Concatenate  NumInputs=3  Mode=Multidimensional array  ConcatenateDimension=2
  Mux4 : Mux  Inputs=3
  Mux5 : Mux  Inputs=3
  Mux6 : Mux  Inputs=3
  Sum1 : Sum  Inputs=|++
  Sum2 : Sum  Inputs=|+-
  Trigonometric Function : Trigonometry  Operator=cos
  Trigonometric Function1 : Trigonometry
  Trigonometric Function2 : Trigonometry  Operator=cos
  Trigonometric Function3 : Trigonometry
  Trigonometric Function4 : Trigonometry  Operator=cos
  Trigonometric Function5 : Trigonometry
  "nT " : Outport
  wires:
  Matrix Concatenate2/1 -> "nT "/1
  theta/1 -> Trigonometric Function1/1, Trigonometric Function/1, Sum2/1, Sum1/1
  Mux6/1 -> Matrix Concatenate2/2
  Mux5/1 -> Matrix Concatenate2/1
  Trigonometric Function5/1 -> Mux6/3
  Trigonometric Function4/1 -> Mux5/3
  Trigonometric Function3/1 -> Mux6/2
  Trigonometric Function2/1 -> Mux5/2
  Trigonometric Function1/1 -> Mux6/1
  Trigonometric Function/1 -> Mux5/1
  Constant4/1 -> Sum1/2, Sum2/2
  Sum1/1 -> Trigonometric Function5/1, Trigonometric Function4/1
  Sum2/1 -> Trigonometric Function3/1, Trigonometric Function2/1
  Constant5/1 -> Mux4/1
  Constant6/1 -> Mux4/2
  Constant7/1 -> Mux4/3
  Mux4/1 -> Matrix Concatenate2/3
